simulink model "VCP_interface_STM32F429_R2018b"  (R2018b)
settings: Solver=FixedStepDiscrete  StartTime=0.0  StopTime=inf  FixedStep=Ts  RelTol=1e-3
InitFcn:
  | datafields_per_usb_transfer = 16;
  | Ts = 10e-3;
undefined symbols (not defined in the file or in its folder): serial
libraries: instrumentlib x3
settings Model: EnablePacing=on  PacingRate=1.100000  Creator=oliver.dieterle  LastModifiedBy=Z0175045
settings DataIOCC: LimitDataPoints=on  SaveFormat=Array
settings OptimizationCC: BlockReduction=off  BooleanDataType=off  LifeSpan=inf
settings DebuggingCC: SaveWithParameterizedLinksMsg=none  UnderspecifiedInitializationDetection=Classic  MergeDetectMultiDrivingBlocksExec=none  SignalResolutionControl=TryResolveAllWithWarning  SFUnexpectedBacktrackingDiag=warning  SFNoUnconditionalDefaultTransitionDiag=warning  SFExecutionAtInitializationDiag=none
settings HardwareCC: ProdBitPerPointer=32  ProdBitPerSizeT=32  ProdBitPerPtrDiffT=32  ProdLargestAtomicFloat=None  ProdIntDivRoundTo=Undefined  ProdEndianess=Unspecified  ProdWordSize=32  ProdHWDeviceType=32-bit Generic  TargetUnknown=on
settings ModelReferenceCC: PropagateSignalLabelsOutOfModel=off
settings SFSimCC: SimUseLocalCustomCode=off
settings RTWCC: RTWUseLocalCustomCode=off
settings CodeAppCC: StateflowObjectComments=on
settings GRTTargetCC: TargetLangStandard=C89/C90 (ANSI)
settings ConfigComp: CovMetricSettings=dw  CovSaveCumulativeToWorkspaceVar=on  CovSaveSingleToWorkspaceVar=on  CovExternalEMLEnable=off  CovSFcnEnable=off

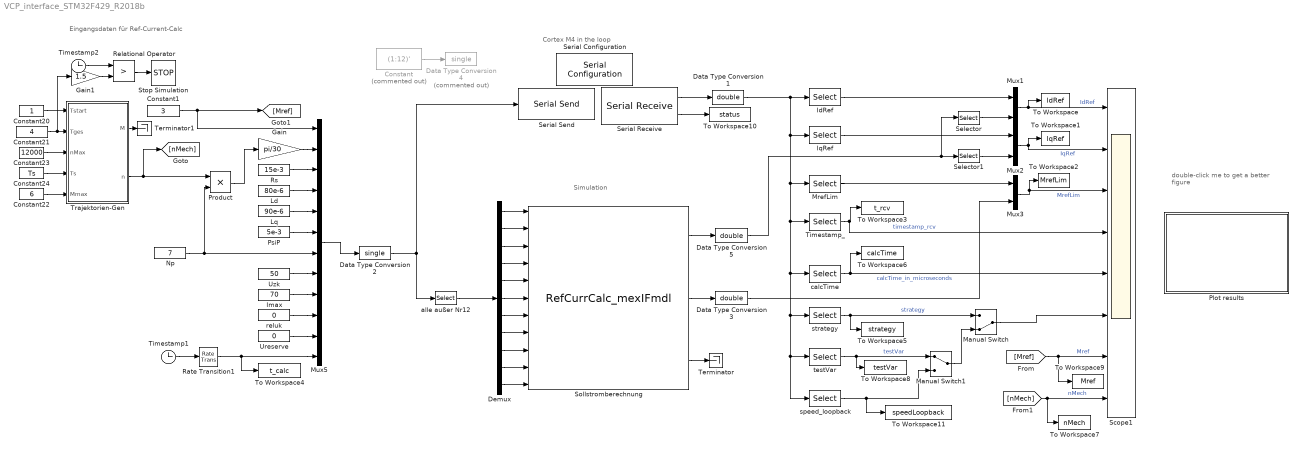
== system VCP_interface_STM32F429_R2018b ==
  note: Simulation
  note: Cortex M4 in the loop
  note: Eingangsdaten für Ref-Current-Calc
  note: double-click me
      | to get a better figure
  Constant : Constant  Commented=on  Value=(1:12)'
  Constant1 : Constant  Value=3
  Constant20 : Constant
  Constant21 : Constant  Value=4
  Constant22 : Constant  Value=6
  Constant23 : Constant  Value=12000
  Constant24 : Constant  Value=Ts
  Data Type Conversion1 : DataTypeConversion  OutDataTypeStr=double
  Data Type Conversion2 : DataTypeConversion  OutDataTypeStr=single
  Data Type Conversion3 : DataTypeConversion  OutDataTypeStr=double
  Data Type Conversion4 : DataTypeConversion  Commented=on  OutDataTypeStr=single
  Data Type Conversion5 : DataTypeConversion  OutDataTypeStr=double
  Demux : Demux  Outputs=11
  Gain : Gain  Gain=pi/30
  Gain1 : Gain  Gain=1.5
  IdRef : Selector  InputPortWidth=datafields_per_usb_transfer  IndexOptions=Index vector (dialog)  Indices=1  OutputSizes=1
  Imax : Constant  Value=70
  IqRef : Selector  InputPortWidth=datafields_per_usb_transfer  IndexOptions=Index vector (dialog)  Indices=2  OutputSizes=1
  Ld : Constant  Value=80e-6
  Lq : Constant  Value=90e-6
  Manual Switch : ManualSwitch  CurrentSetting=0
  Manual Switch1 : ManualSwitch
  MrefLim : Selector  InputPortWidth=datafields_per_usb_transfer  IndexOptions=Index vector (dialog)  Indices=3  OutputSizes=1
  Mux1 : Mux  Inputs=2
  Mux2 : Mux  Inputs=2
  Mux3 : Mux  Inputs=2
  Mux5 : Mux  Inputs=12
  Np : Constant  Value=7
  Plot results : Subsystem
      settings: OpenFcn=plot_results;
  Product : Product
  PsiP : Constant  Value=5e-3
  Rate Transition1 : RateTransition  OutPortSampleTime=Ts
  Relational Operator : RelationalOperator  Operator=>  OutDataTypeStr=boolean  RndMeth=Simplest
  Rs : Constant  Value=15e-3
  Scope1 : Scope  NumInputPorts=8
  Selector : Selector  InputPortWidth=2  IndexOptions=Index vector (dialog)  Indices=1  OutputSizes=1
  Selector1 : Selector  InputPortWidth=2  IndexOptions=Index vector (dialog)  Indices=2  OutputSizes=1
  Serial Configuration : instrumentlib/Serial Configuration  Priority=-200000  ComPortMenu=COM8  ComPort=COM8  ObjConstructor=serial('COM8');  BaudRate=256000  DataBits=8  Parity=none  StopBits=1  FlowControl=none  Timeout=3  ByteOrder=LittleEndian
  Serial Receive : instrumentlib/Serial Receive  ComPortMenu=COM8  ComPort=COM8  ObjConstructor=serial('COM8');  Header=HEAD  Terminator=<none>  DataSize="[16   1]"  DataType=single  EnableBlockingMode=off  ActionDataUnavailable=Output last received value  CustomValue=0  SampleTime=Ts
  Serial Send : instrumentlib/Serial Send  ComPortMenu=COM8  ComPort=COM8  ObjConstructor=serial('COM8');  Header=HEAD  Terminator=<none>  EnableBlockingMode=off
  Sollstromberechnung : S-Function  FunctionName=RefCurrCalc_mexIFmdl  SFunctionModules='D:\Programming\CCode\Sollstromberechnung\Implementierung_v03\Test_in_Matlab\RefCurrentCalculation_main_Full'  SFunctionDeploymentMode=off  EnableBusSupport=off
      mask Display:
      | text(0.3,0.97,'Sollstromberechnung')
      | 
      | port_label('input', 1, 'Mref [Nm]')
      | port_label('input', 2, 'omEl [rad/s]')
      | port_label('input', 3, 'Rs [Ohm]')
      | port_label('input', 4, 'Ld [H]')
      | port_label('input', 5, 'Lq [H]')
      | port_label('input', 6, 'PsiP [Vs]')
      | port_label('input', 7, 'Np [1]')
      | port_label('input', 8, 'Uzk [V]')
      | port_label('input', 9, 'Imax [A]')
      | port_label('input', 10, 'reluk [V]')
      | port_label('input', 11, 'Ureserve [V]')
      | 
      | port_label('output', 1, 'IdqRef [A]')
      | port_label('output', 2, 'MrefLim [Nm]')
      | port_label('output', 3, 'diag [-]')
  Stop Simulation : Stop
  Terminator : Terminator
  Terminator1 : Terminator
  Timestamp1 : Clock
  Timestamp2 : Clock
  Timestamp_ : Selector  InputPortWidth=datafields_per_usb_transfer  IndexOptions=Index vector (dialog)  Indices=4  OutputSizes=1
  To Workspace : ToWorkspace  VariableName=IdRef  SampleTime=Ts
  To Workspace1 : ToWorkspace  VariableName=IqRef  SampleTime=Ts
  To Workspace10 : ToWorkspace  VariableName=status  SaveFormat=Timeseries  SampleTime=Ts
  To Workspace11 : ToWorkspace  VariableName=speedLoopback  SampleTime=Ts
  To Workspace2 : ToWorkspace  VariableName=MrefLim  SampleTime=Ts
  To Workspace3 : ToWorkspace  VariableName=t_rcv  SampleTime=Ts
  To Workspace4 : ToWorkspace  VariableName=t_calc  SampleTime=Ts
  To Workspace5 : ToWorkspace  VariableName=strategy  SampleTime=Ts
  To Workspace6 : ToWorkspace  VariableName=calcTime  SampleTime=Ts
  To Workspace7 : ToWorkspace  VariableName=nMech  SampleTime=Ts
  To Workspace8 : ToWorkspace  VariableName=testVar  SampleTime=Ts
  To Workspace9 : ToWorkspace  VariableName=Mref  SampleTime=Ts
  Trajektorien-Gen : MATLAB Function  TreatAsAtomicUnit=on  SystemSampleTime=Ts
  Ureserve : Constant  Value=0
  Uzk : Constant  Value=50
  alle außer Nr12 : Selector  InputPortWidth=12  IndexOptions=Index vector (dialog)  Indices=(1:11)  OutputSizes=1
  calcTime : Selector  InputPortWidth=datafields_per_usb_transfer  IndexOptions=Index vector (dialog)  Indices=5  OutputSizes=1
  reluk : Constant  Value=0
  speed_loopback : Selector  InputPortWidth=datafields_per_usb_transfer  IndexOptions=Index vector (dialog)  Indices=8  OutputSizes=1
  strategy : Selector  InputPortWidth=datafields_per_usb_transfer  IndexOptions=Index vector (dialog)  Indices=7  OutputSizes=1
  testVar : Selector  InputPortWidth=datafields_per_usb_transfer  IndexOptions=Index vector (dialog)  Indices=6  OutputSizes=1
  wires:
  Data Type Conversion2/1 -> Serial Send/1, alle außer Nr12/1
  Serial Receive/2 -> To Workspace10/1
  Serial Receive/1 -> Data Type Conversion1/1
  Mux1/1 -> To Workspace/1, Scope1/1  "IdRef"
  Mux2/1 -> Scope1/2, To Workspace1/1  "IqRef"
  Mux3/1 -> To Workspace2/1, Scope1/3  "MrefLim"
  IdRef/1 -> Mux1/1
  IqRef/1 -> Mux2/1
  MrefLim/1 -> Mux3/1
  Selector/1 -> Mux1/2
  Selector1/1 -> Mux2/2
  calcTime/1 -> To Workspace6/1, Scope1/5  "calcTime_in_microseconds"
  Demux/2 -> Sollstromberechnung/2
  Demux/1 -> Sollstromberechnung/1
  Demux/4 -> Sollstromberechnung/4
  Demux/6 -> Sollstromberechnung/6
  Demux/7 -> Sollstromberechnung/7
  Demux/8 -> Sollstromberechnung/8
  Demux/9 -> Sollstromberechnung/9
  Demux/10 -> Sollstromberechnung/10
  Demux/5 -> Sollstromberechnung/5
  Demux/3 -> Sollstromberechnung/3
  Demux/11 -> Sollstromberechnung/11
  Constant1/1 -> Mux5/1, [Mref]
  Rs/1 -> Mux5/3
  PsiP/1 -> Mux5/6
  Uzk/1 -> Mux5/8
  Imax/1 -> Mux5/9
  reluk/1 -> Mux5/10
  Ureserve/1 -> Mux5/11
  Sollstromberechnung/1 -> Data Type Conversion5/1
  Sollstromberechnung/2 -> Data Type Conversion3/1
  Trajektorien-Gen/2(n) -> Product/1, [nMech]
  Timestamp1/1 -> Rate Transition1/1
  alle außer Nr12/1 -> Demux/1
  Data Type Conversion1/1 -> IdRef/1, IqRef/1, speed_loopback/1, testVar/1, strategy/1, calcTime/1, Timestamp_/1, MrefLim/1
  Data Type Conversion3/1 -> Mux3/2
  Data Type Conversion5/1 -> Selector/1, Selector1/1
  Constant20/1 -> Trajektorien-Gen/1(Tstart)
  Constant24/1 -> Trajektorien-Gen/4(Ts)
  Constant23/1 -> Trajektorien-Gen/3(nMax)
  Constant22/1 -> Trajektorien-Gen/5(Mmax)
  Gain/1 -> Mux5/2
  Relational Operator/1 -> Stop Simulation/1
  Timestamp2/1 -> Relational Operator/1
  Mux5/1 -> Data Type Conversion2/1
  Rate Transition1/1 -> To Workspace4/1, Mux5/12
  Constant21/1 -> Gain1/1, Trajektorien-Gen/2(Tges)
  Lq/1 -> Mux5/5
  Ld/1 -> Mux5/4
  Timestamp_/1 -> Scope1/4, To Workspace3/1  "timestamp_rcv"
  Sollstromberechnung/3 -> Terminator/1
  strategy/1 -> Manual Switch/1, To Workspace5/1  "strategy"
  [nMech] -> Scope1/8, To Workspace7/1  "nMech"
  [Mref] -> Scope1/7, To Workspace9/1  "Mref"
  Gain1/1 -> Relational Operator/2
  testVar/1 -> Manual Switch1/1, To Workspace8/1  "testVar"
  speed_loopback/1 -> Manual Switch1/2, To Workspace11/1
  Manual Switch/1 -> Scope1/6
  Constant/1 -> Data Type Conversion4/1
  Manual Switch1/1 -> Manual Switch/2
  Trajektorien-Gen/1(M) -> Terminator1/1
  Np/1 -> Mux5/7, Product/2
  Product/1 -> Gain/1

== system VCP_interface_STM32F429_R2018b/Plot results ==

== matlab function VCP_interface_STM32F429_R2018b/Trajektorien-Gen ==
  data: Tstart input; M output; Tges input; nMax input; Ts input; Mmax input; n output
function [M,n] = fcn(Tstart,Tges,nMax,Ts,Mmax)

persistent t

if(isempty(t)) t = 0; end

Tges = Tges/2;

t = t+Ts;
dn = nMax/Tges;


M = 0;
n = 0;

t_sin = t-Tstart;
    
if(t > Tstart+2*Tges)
    M = 0;
    n = 0;    
elseif(t > Tstart+2*Tges)
    M = Mmax*sin(2*pi*t_sin/(2*Tges));
    n = -dn*(t-(Tstart+2*Tges));
elseif(t > Tstart+Tges)
    M = Mmax*sin(2*pi*t_sin/(2*Tges));
    n = nMax - dn*(t-(Tstart+Tges));
elseif(t > Tstart)
    M = Mmax*sin(2*pi*t_sin/(2*Tges));
    n = dn*(t-Tstart);
end

end
